simulink model "sf_yoyo"  (Simulink 6.0)
settings: Solver=ode23  StartTime=0.0  StopTime=500  FixedStep=1  RelTol=1e-3
settings Model: CovMetricSettings=dcmtr  Creator=The MathWorks Inc.  LastModifiedBy=batserve  ExtModeTrigMode=oneshot  ExtModeArmWhenConnect=off  ExtModeAutoUpdateStatusClock=off  BufferReuse=off
settings DataIOCC: LimitDataPoints=off  SaveOutput=off  SaveTime=off
settings OptimizationCC: BlockReduction=off  BooleanDataType=off  OptimizeBlockIOStorage=off  BufferReuse=off  ExpressionFolding=off  LocalBlockOutputs=off
settings DebuggingCC: CheckExecutionContextPreStartOutputMsg=on  CheckExecutionContextRuntimeOutputMsg=on  SolverPrmCheckMsg=none
settings HardwareCC: TargetUnknown=on

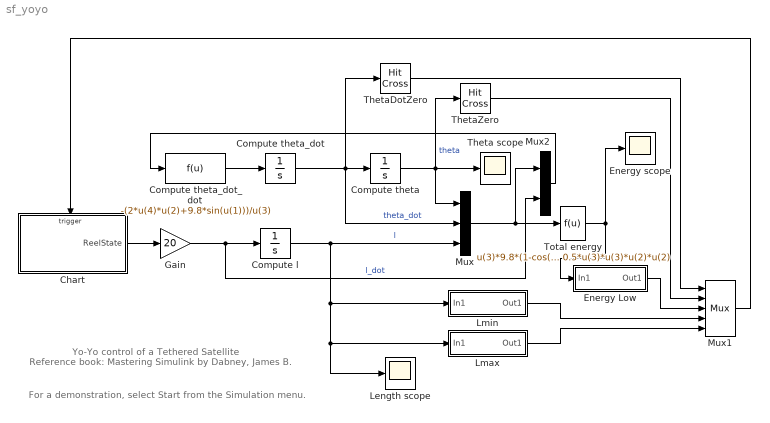
== system sf_yoyo ==
  note: Yo-Yo control of a Tethered Satellite
  note: For a demonstration, select Start from the Simulation menu.
  note: Reference book: Mastering Simulink by Dabney, James B.
  Chart : Stateflow chart  TreatAsAtomicUnit=on  PropExecContextAcrossSSBoundary=on
  Compute theta : Integrator  InitialCondition=0.16
  Compute theta_dot : Integrator
  Compute theta_dot_dot : Fcn  Expr=-(2*u(4)*u(2)+9.8*sin(u(1)))/u(3)
  Compute l : Integrator  InitialCondition=100  UpperSaturationLimit=105  LowerSaturationLimit=95
  Energy scope : Scope
      settings: TimeRange=500  YMin=0  YMax=15  SaveName=EnergyTraj
  Energy Low : Subsystem  PropExecContextAcrossSSBoundary=on  mask{th=0.001}
      mask prompts: th "Lower Limit"
      mask Display: disp('y = (u <= lim)')
  Gain : Gain  Gain=20  SaturateOnIntegerOverflow=on
  Length scope : Scope
      settings: TimeRange=500  YMin=90  YMax=110  SaveName=LengthTraj
  Lmax : Subsystem  PropExecContextAcrossSSBoundary=on  mask{th=105}
      mask prompts: th "Upper Limit"
      mask Display: disp('y = (u >= lim)')
  Lmin : Subsystem  PropExecContextAcrossSSBoundary=on  mask{th=95}
      mask prompts: th "Lower Limit"
      mask Display: disp('y = (u <= lim)')
  Mux : Mux  Inputs=3
  Mux1 : Mux  Inputs=5
  Mux2 : Mux  Inputs=2
  Theta scope : Scope
      settings: TimeRange=500  YMin=-0.2  YMax=0.2  SaveName=ThetaTraj
  ThetaDotZero : HitCross
  ThetaZero : HitCross
  "Total energy " : Fcn  Expr=u(3)*9.8*(1-cos(u(1))) + 0.5*u(3)*u(3)*u(2)*u(2)
  wires:
  Compute theta_dot_dot/1 -> Compute theta_dot/1
  Chart/1(ReelState) -> Gain/1
  Compute theta_dot/1 -> Compute theta/1, ThetaDotZero/1, Mux/2  "theta_dot"
  Gain/1 -> Compute l/1, Mux2/2  "l_dot"
  Compute theta/1 -> ThetaZero/1, Theta scope/1, Mux/1  "theta"
  Mux1/1 -> Chart/Trigger
  Mux/1 -> "Total energy "/1, Mux2/1
  Energy Low/1(Out1) -> Mux1/3
  ThetaZero/1 -> Mux1/2
  ThetaDotZero/1 -> Mux1/1
  Compute l/1 -> Mux/3, Length scope/1, Lmax/1(In1), Lmin/1(In1)  "l"
  Mux2/1 -> Compute theta_dot_dot/1
  "Total energy "/1 -> Energy scope/1, Energy Low/1(In1)
  Lmin/1(Out1) -> Mux1/4
  Lmax/1(Out1) -> Mux1/5

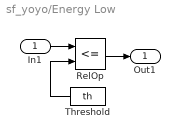
== system sf_yoyo/Energy Low ==
  In1 : Inport  Port=1  LatchInput=off
  RelOp : RelationalOperator  Operator=<=
  Threshold : Constant  Orientation=left  Value=th
  Out1 : Outport
  wires:
  Threshold/1 -> RelOp/2
  In1/1 -> RelOp/1
  RelOp/1 -> Out1/1

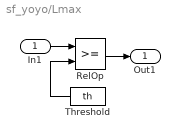
== system sf_yoyo/Lmax ==
  In1 : Inport  Port=1  LatchInput=off
  RelOp : RelationalOperator
  Threshold : Constant  Orientation=left  Value=th
  Out1 : Outport
  wires:
  Threshold/1 -> RelOp/2
  In1/1 -> RelOp/1
  RelOp/1 -> Out1/1

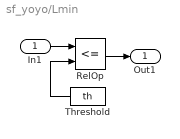
== system sf_yoyo/Lmin ==
  In1 : Inport  Port=1  LatchInput=off
  RelOp : RelationalOperator  Operator=<=
  Threshold : Constant  Orientation=left  Value=th
  Out1 : Outport
  wires:
  RelOp/1 -> Out1/1
  In1/1 -> RelOp/1
  Threshold/1 -> RelOp/2

== stateflow chart Chart ==
  settings: sampleTime=1
  state Active
    state ReelMoving
      /* example of Moore type action */
      exit: ReelState = 0;
      state ReelOut
        entry: ReelState = 1;
      state ReelIn
        entry:ReelState= -1;
    state ReelStop
    (default) -> ReelStop
    ReelStop -> ReelOut : ThetaZero
    ReelOut -> ReelStop : Lmax
    ReelIn -> ReelStop : Lmin
    ReelStop -> ReelIn : ThetaDotZero
  state Inactive
  (default) -> Active : {ReelState = 0;} /* example of Mealy type action */
  Active -> Inactive : EnergyLow
  data: ReelState output double size=1
  events: ThetaDotZero input EITHER_EDGE_EVENT; ThetaZero input EITHER_EDGE_EVENT; EnergyLow input EITHER_EDGE_EVENT; Lmin input EITHER_EDGE_EVENT; Lmax input EITHER_EDGE_EVENT
